simulink model "VendingMachine_MealySematic"  (R2020a)
settings: Solver=VariableStepAuto  StartTime=0.0  StopTime=10.0  RelTol=1e-3
settings Model: Creator=DELL  LastModifiedBy=DELL

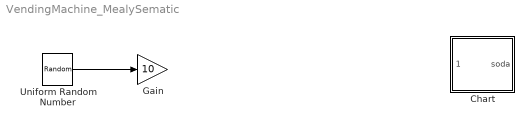
== system VendingMachine_MealySematic ==
  Chart : Stateflow chart  TreatAsAtomicUnit=on
  Gain : Gain  Gain=10
  Uniform Random Number : UniformRandomNumber  Minimum=0  Maximum=2  SampleTime=0.1
  wires:
  Uniform Random Number/1 -> Gain/1

== stateflow chart VendingMachine_MealySematic/Chart ==
  state got_0Rs
  state got_10Rs
  state got_20Rs
  (default) -> got_0Rs
  got_0Rs -> got_10Rs [order 1] : [money == 10]{soda = 0;}
  got_10Rs -> got_0Rs [order 2] : [money == 20]{soda = 1;}
  got_0Rs -> got_20Rs [order 2] : [money == 20]{soda = 0;}
  got_20Rs -> got_0Rs [order 1] : [money == 10]{soda = 1;}
  got_20Rs -> got_10Rs [order 2] : [money == 20]{soda = 1;}
  got_10Rs -> got_20Rs [order 1] : [money == 10]{soda = 0;}
  data: money input; soda output
